simulink model "Problem3_AutomaticTransmissionControl"  (R2020b)
settings: Solver=ode5  StartTime=0.0  StopTime=50  FixedStep=0.04  RelTol=1e-3
PreLoadFcn:
  | clearvars
  | load('vehicleData.mat')
StartFcn:
  | cput= cputime;
StopFcn:
  | disp("CPU Time Elapsed"); cputime-cput
undefined symbols (not defined in the file): DOWN_TABLE, DOWN_TH_BP, EMAP, Iei, Iv, Kfactor, N20, NE_VEC, Rfd, rload0, rload2, Rw, sigbuilder_block, speedratio, TH_VEC, Torkratio, UP_TABLE, UP_TH_BP
CloseFcn:
  | clearvars
settings Model: DataDictionary=Data.sldd  Creator=vigne  LastModifiedBy=prabhudevmaddipudi

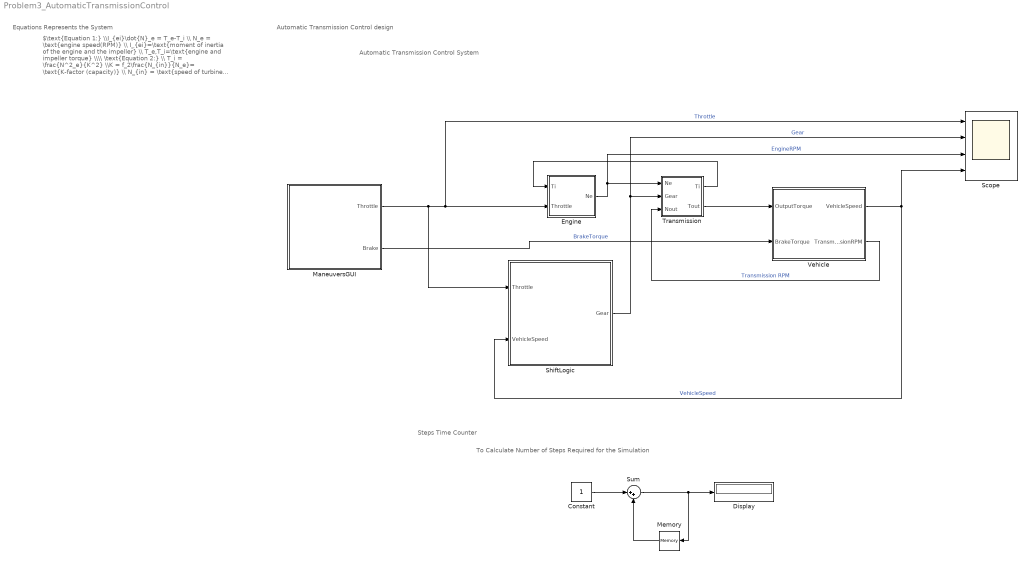
== system Problem3_AutomaticTransmissionControl ==
  note: Equations Represents the System
  note: $\text{Equation 1:} \\I_{ei}\dot{N}_e = T_e-T_i \\ N_e = \text{engine speed(RPM)} \\ I_{ei}=\text{moment of inertia of the engine and the impeller} \\ T_e,T_i=\text{engine and impeller torque} \\\\ \text{Equation 2:} \\ T_i = \frac{N^2_e}{K^2} \\K = f_2\frac{N_{in}}{N_e}= \text{K-factor (capacity)} \\ N_{in} = \text{speed of turbine (torque converter output)} \\ R_{TQ}= f_3\frac{N_{in}}{N_e}= \text{torque ratio} \\\\ \text{Equation 3:} \\ R_{TR}= f_4(gear) = \text{transmission ratio} \\ T_{out}=R_{TR}T_{in} \\ N_{in} = R_{TR}N_{out} \\ T_{in}, T_{out}= \text{transmission input and output torques} \\ N_{in}, N_{out} = \text{transmission input and output speed (RPM)} \\\\ \text{Equation 4:} \\ I_v\dot{N}_w= R_{fd}(T_{out}-T_{load}) \\ I_v= \text{vehicle inertia} \\ N_w = \text{wheel speed(RPM)} \\ R_{fd}= \text{final drive ratio} \\ T_{load}=f_s(N_w)=\text{load torque} \\\\ \text{Equation 5:} \\ T_{load}=sgn\left(mph\right)\left(R_{load0}+R_{load2}mph^2+T_{brake}\right) \\ R_{load0},R_{load2}= \text{friction and aerodynamic drag coefficients} \\ T_{load},T_{brake} = \text{load and break torque} \\ mph = \text{vehicle linear velocity}$
  note: Automatic Transmission Control design
  note: Steps Time Counter
  note: To Calculate Number of Steps Required for the Simulation
  note: Automatic Transmission Control System
  Constant : Constant
  Display : Display
  Engine : Subsystem
  ManeuversGUI : Subsystem  Tag=STV Subsys  LoadFcn=sigbuilder_block('load');  StartFcn=sigbuilder_block('start');  StopFcn=sigbuilder_block('stop');  ClipboardFcn=sigbuilder_block('clipboard');  mask(Sigbuilder block){tuvar=[0:10]}
      mask help: Sigbuilder GUI
      mask init:
      | tuvar = sigbuilder_block('maskInit');
      settings: CopyFcn=sigbuilder_block('copy');  DeleteFcn=sigbuilder_block('delete');  ModelCloseFcn=sigbuilder_block('modelClose');  PreSaveFcn=sigbuilder_block('preSave');  PauseFcn=sigbuilder_block('pause')  ContinueFcn=sigbuilder_block('continue')  NameChangeFcn=sigbuilder_block('namechange');  OpenFcn=sigbuilder_block('open',[6 22.5 1012.5 455.25 ]);  CloseFcn=sigbuilder_block('close');
      mask Display: plot(0, 0, 100, 100,[2, 2, 32, 32, 2], [68, 8, 8, 68, 68],[32, 2], [38, 38], [32, 19, 2],[53, 60, 44], [32, 17, 17, 2],[16, 16, 31, 31]);txt = getActiveGroup(gcbh);text(2, 100, txt,'verticalAlignment', 'top');
  Memory : Memory
  Scope : Scope  NumInputPorts=4
  ShiftLogic : Stateflow chart  TreatAsAtomicUnit=on
  Sum : Sum  Inputs=|++
  Transmission : Subsystem
  Vehicle : Subsystem
  wires:
  Transmission/2(Tout) -> Vehicle/1(OutputTorque)
  Transmission/1(Ti) -> Engine/1(Ti)
  Engine/1(Ne) -> Scope/3, Transmission/1(Ne)  "EngineRPM"
  ManeuversGUI/1(Throttle) -> ShiftLogic/1(Throttle), Scope/1, Engine/2(Throttle)  "Throttle"
  Vehicle/1(VehicleSpeed) -> Scope/4, ShiftLogic/2(VehicleSpeed)  "VehicleSpeed"
  Vehicle/2(TransmissionRPM) -> Transmission/3(Nout)  "Transmission RPM"
  ManeuversGUI/2(Brake) -> Vehicle/2(BrakeTorque)  "BrakeTorque"
  ShiftLogic/1(Gear) -> Scope/2, Transmission/2(Gear)  "Gear"
  Constant/1 -> Sum/1
  Sum/1 -> Memory/1, Display/1
  Memory/1 -> Sum/2

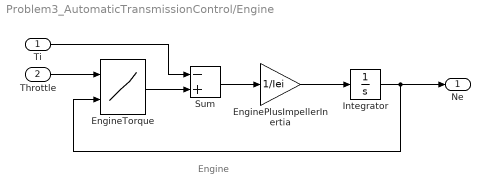
== system Problem3_AutomaticTransmissionControl/Engine ==
  note: Engine
  Ti : Inport  Unit=ft*lbf@torque
  Throttle : Inport  Port=2  Unit=%
  EnginePlusImpellerInertia : Gain  Gain=1/Iei  SaturateOnIntegerOverflow=on  OutDataTypeStr=Inherit: Same as input  ParamDataTypeStr=Inherit: Same as input
  EngineTorque : Lookup_n-D  BreakpointsForDimension1=TH_VEC  BreakpointsForDimension2=NE_VEC  Table=EMAP  InputSameDT=on
      settings: InputPortMap=u0,u1
  Integrator : Integrator  InitialCondition=1000  LimitOutput=on  UpperSaturationLimit=6000  LowerSaturationLimit=600  ZeroCross=off
  Sum : Sum  Inputs=-+  InputSameDT=on  SaturateOnIntegerOverflow=on  OutDataTypeStr=Inherit: Same as first input
  Ne : Outport  Unit=rpm  VectorParamsAs1DForOutWhenUnconnected=off
  wires:
  EnginePlusImpellerInertia/1 -> Integrator/1
  EngineTorque/1 -> Sum/2
  Ti/1 -> Sum/1
  Integrator/1 -> EngineTorque/2, Ne/1
  Throttle/1 -> EngineTorque/1
  Sum/1 -> EnginePlusImpellerInertia/1

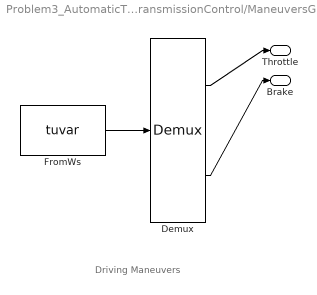
== system Problem3_AutomaticTransmissionControl/ManeuversGUI ==
  note: Driving Maneuvers
  Demux : Demux  Tag=STV Demux  Outputs=2
      settings: DisplayOption=none
  FromWs : FromWorkspace  Tag=STV FromWs  VariableName=tuvar  ZeroCross=off
      SigBuilderData=|
      | dataSet(1).timeRange = [0 50]
      | dataSet(1).name = 'Passing Maneuver'
      | dataSet(2).timeRange = [0 50]
      | dataSet(2).name = 'Gradual Acceleration'
      | dataSet(3).timeRange = [0 50]
      | dataSet(3).name = 'Hard braking'
      | dataSet(4).timeRange = [0 50]
      | dataSet(4).name = 'Coasting'
      | sbobj.Groups(1).Name = 'Passing Maneuver'
      | sbobj.Groups(1).Signals(1).Name = 'Throttle'
      | sbobj.Groups(1).Signals(1).XData = [0 14.9 15 27.55 33.45 40 50]
      | sbobj.Groups(1).Signals(1).YData = [60 40 100 1 80 41 100]
      | sbobj.Groups(1).Signals(2).Name = 'Brake'
      | sbobj.Groups(1).Signals(2).XData = [0 44.95 44.95 50]
      | sbobj.Groups(1).Signals(2).YData = [0 0 -0.55 -0.55]
      | sbobj.Groups(1).TimeRange = [0 50]
      | sbobj.Groups(2).Name = 'Gradual Acceleration'
      | sbobj.Groups(2).Signals(1).Name = 'Throttle'
      | sbobj.Groups(2).Signals(1).XData = [0 50]
      | sbobj.Groups(2).Signals(1).YData = [13.4 24]
      | sbobj.Groups(2).Signals(2).Name = 'Brake'
      | sbobj.Groups(2).Signals(2).XData = [0 50]
      | sbobj.Groups(2).Signals(2).YData = [0 0]
      | sbobj.Groups(2).TimeRange = [0 50]
      | sbobj.Groups(3).Name = 'Hard braking'
      | sbobj.Groups(3).Signals(1).Name = 'Throttle'
      | sbobj.Groups(3).Signals(1).XData = [0 5.1 5.1 50]
      | sbobj.Groups(3).Signals(1).YData = [50 50 1 1]
      | sbobj.Groups(3).Signals(2).Name = 'Brake'
      | sbobj.Groups(3).Signals(2).XData = [0 10 10 50]
      | sbobj.Groups(3).Signals(2).YData = [0 0 325 325]
      | sbobj.Groups(3).TimeRange = [0 50]
      | sbobj.Groups(4).Name = 'Coasting'
      | sbobj.Groups(4).Signals(1).Name = 'Throttle'
      | sbobj.Groups(4).Signals(1).XData = [0 4.8 4.8 50]
      | sbobj.Groups(4).Signals(1).YData = [80 80 1 1]
      | sbobj.Groups(4).Signals(2).Name = 'Brake'
      | sbobj.Groups(4).Signals(2).XData = [0 50]
      | sbobj.Groups(4).Signals(2).YData = [0 0]
      | sbobj.Groups(4).TimeRange = [0 50]
  Throttle : Outport  Tag=STV Outport  VectorParamsAs1DForOutWhenUnconnected=off
  Brake : Outport  Tag=STV Outport  Port=2  VectorParamsAs1DForOutWhenUnconnected=off
  wires:
  FromWs/1 -> Demux/1
  Demux/1 -> Throttle/1
  Demux/2 -> Brake/1

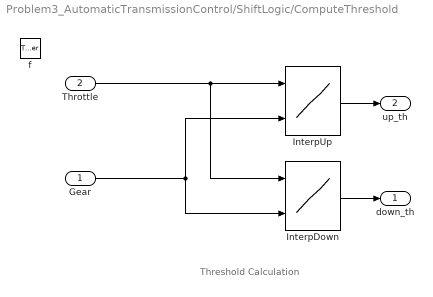
== system Problem3_AutomaticTransmissionControl/ShiftLogic/ComputeThreshold ==
  note: Threshold Calculation
  Gear : Inport
  Throttle : Inport  Port=2
  f : TriggerPort  TriggerType=function-call  VariantControl=(inherit)
      settings: CopyFcn=Stateflow.SLINSF.SimulinkMan.removeBlockPreDeleteFcn  PreDeleteFcn=Stateflow.SLINSF.SimulinkMan.unsafePredeleteFcn
  InterpDown : Lookup_n-D  BreakpointsForDimension1=DOWN_TH_BP  BreakpointsForDimension2=[1:4]  Table=DOWN_TABLE  OutDataTypeStr=double  LockScale=on
      settings: InputPortMap=u0,u1
  InterpUp : Lookup_n-D  BreakpointsForDimension1=UP_TH_BP  BreakpointsForDimension2=[1:4]  Table=UP_TABLE  OutDataTypeStr=double  LockScale=on
      settings: InputPortMap=u0,u1
  down_th : Outport  InitialOutput=0  VectorParamsAs1DForOutWhenUnconnected=off
  up_th : Outport  Port=2  InitialOutput=0  VectorParamsAs1DForOutWhenUnconnected=off
  wires:
  InterpUp/1 -> up_th/1
  InterpDown/1 -> down_th/1
  Throttle/1 -> InterpDown/1, InterpUp/1
  Gear/1 -> InterpDown/2, InterpUp/2

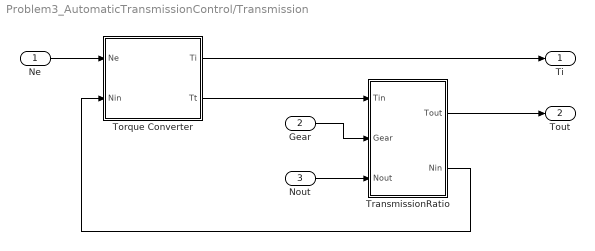
== system Problem3_AutomaticTransmissionControl/Transmission ==
  Ne : Inport  Unit=rpm
  Gear : Inport  Port=2  Unit=1
  Nout : Inport  Port=3  Unit=rpm
  Torque Converter : Subsystem
  TransmissionRatio : Subsystem
  Ti : Outport  Unit=ft*lbf@torque  VectorParamsAs1DForOutWhenUnconnected=off
  Tout : Outport  Port=2  Unit=ft*lbf@torque  VectorParamsAs1DForOutWhenUnconnected=off
  wires:
  Torque Converter/2(Tt) -> TransmissionRatio/1(Tin)
  Ne/1 -> Torque Converter/1(Ne)
  Torque Converter/1(Ti) -> Ti/1
  Nout/1 -> TransmissionRatio/3(Nout)
  Gear/1 -> TransmissionRatio/2(Gear)
  TransmissionRatio/2(Nin) -> Torque Converter/2(Nin)
  TransmissionRatio/1(Tout) -> Tout/1

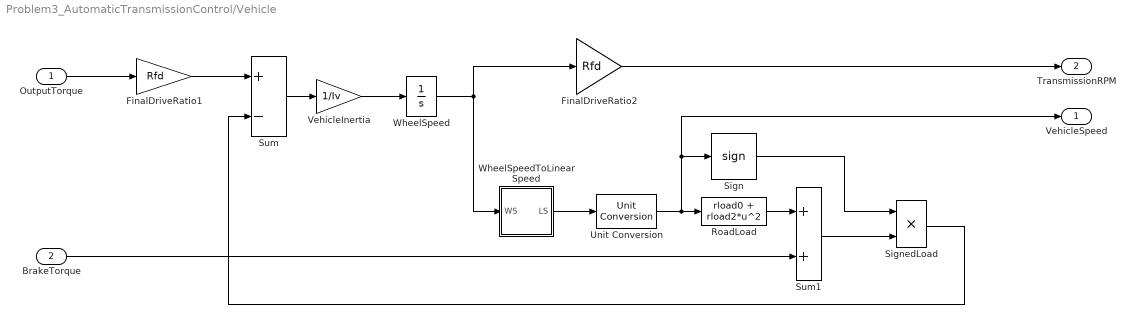
== system Problem3_AutomaticTransmissionControl/Vehicle ==
  OutputTorque : Inport  Unit=ft*lbf@torque
  BrakeTorque : Inport  Port=2  Unit=ft*lbf@torque
  FinalDriveRatio1 : Gain  Gain=Rfd  SaturateOnIntegerOverflow=on  OutDataTypeStr=Inherit: Same as input  ParamDataTypeStr=Inherit: Same as input
  FinalDriveRatio2 : Gain  Gain=Rfd  SaturateOnIntegerOverflow=on  OutDataTypeStr=Inherit: Same as input  ParamDataTypeStr=Inherit: Same as input
  RoadLoad : Fcn  Expr=rload0 + rload2*u^2
  Sign : Signum
  SignedLoad : Product  InputSameDT=on  SaturateOnIntegerOverflow=on  OutDataTypeStr=Inherit: Same as first input
  Sum : Sum  Inputs=+-  InputSameDT=on  SaturateOnIntegerOverflow=on  OutDataTypeStr=Inherit: Same as first input
  Sum1 : Sum  InputSameDT=on  SaturateOnIntegerOverflow=on  OutDataTypeStr=Inherit: Same as first input
  Unit Conversion : UnitConversion
  VehicleInertia : Gain  Gain=1/Iv  SaturateOnIntegerOverflow=on  OutDataTypeStr=Inherit: Same as input  ParamDataTypeStr=Inherit: Same as input
  WheelSpeed : Integrator  InitialCondition=N20/Rfd  ZeroCross=off
  WheelSpeedToLinearSpeed : Subsystem
  VehicleSpeed : Outport  Unit=mph  VectorParamsAs1DForOutWhenUnconnected=off
  TransmissionRPM : Outport  Port=2  Unit=rpm  VectorParamsAs1DForOutWhenUnconnected=off
  wires:
  FinalDriveRatio2/1 -> TransmissionRPM/1
  Unit Conversion/1 -> VehicleSpeed/1, Sign/1, RoadLoad/1
  OutputTorque/1 -> FinalDriveRatio1/1
  Sum1/1 -> SignedLoad/2
  WheelSpeed/1 -> FinalDriveRatio2/1, WheelSpeedToLinearSpeed/1(WS)
  WheelSpeedToLinearSpeed/1(LS) -> Unit Conversion/1
  Sum/1 -> VehicleInertia/1
  Sign/1 -> SignedLoad/1
  BrakeTorque/1 -> Sum1/2
  SignedLoad/1 -> Sum/2
  RoadLoad/1 -> Sum1/1
  VehicleInertia/1 -> WheelSpeed/1
  FinalDriveRatio1/1 -> Sum/1

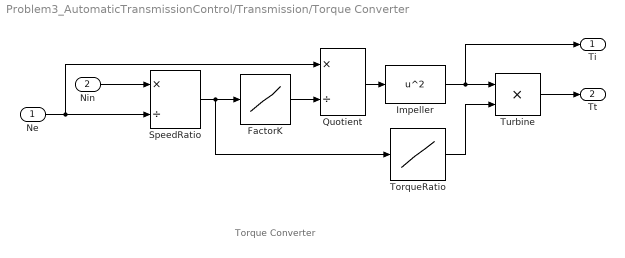
== system Problem3_AutomaticTransmissionControl/Transmission/Torque Converter ==
  note: Torque Converter
  Ne : Inport
  Nin : Inport  Port=2
  FactorK : Lookup_n-D  NumberOfTableDimensions=1  BreakpointsForDimension1=speedratio  Table=Kfactor  SaturateOnIntegerOverflow=on  InputSameDT=on
  Impeller : Fcn  Expr=u^2
  Quotient : Product  Inputs=*/  InputSameDT=on  SaturateOnIntegerOverflow=on  OutDataTypeStr=Inherit: Same as first input
  SpeedRatio : Product  Inputs=*/  InputSameDT=on  SaturateOnIntegerOverflow=on  OutDataTypeStr=Inherit: Same as first input
  TorqueRatio : Lookup_n-D  NumberOfTableDimensions=1  BreakpointsForDimension1=speedratio  Table=Torkratio  SaturateOnIntegerOverflow=on  InputSameDT=on
  Turbine : Product  InputSameDT=on  SaturateOnIntegerOverflow=on  OutDataTypeStr=Inherit: Same as first input
  Ti : Outport  VectorParamsAs1DForOutWhenUnconnected=off
  Tt : Outport  Port=2  VectorParamsAs1DForOutWhenUnconnected=off
  wires:
  Quotient/1 -> Impeller/1
  TorqueRatio/1 -> Turbine/2
  FactorK/1 -> Quotient/2
  Ne/1 -> SpeedRatio/2, Quotient/1
  Nin/1 -> SpeedRatio/1
  SpeedRatio/1 -> TorqueRatio/1, FactorK/1
  Impeller/1 -> Ti/1, Turbine/1
  Turbine/1 -> Tt/1

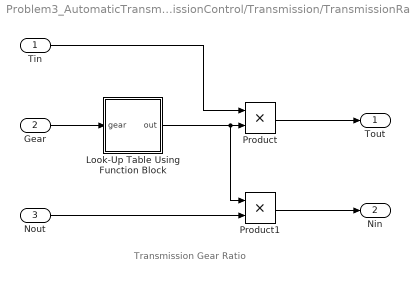
== system Problem3_AutomaticTransmissionControl/Transmission/TransmissionRatio ==
  note: Transmission Gear Ratio
  Tin : Inport  Unit=ft*lbf@torque
  Gear : Inport  Port=2  Unit=1
  Nout : Inport  Port=3  Unit=rpm
  Look-Up Table Using Function Block : MATLAB Function  TreatAsAtomicUnit=on
  Product : Product  InputSameDT=on  SaturateOnIntegerOverflow=on  OutDataTypeStr=Inherit: Same as first input
  Product1 : Product  InputSameDT=on  SaturateOnIntegerOverflow=on  OutDataTypeStr=Inherit: Same as first input
  Tout : Outport  Unit=ft*lbf@torque  VectorParamsAs1DForOutWhenUnconnected=off
  Nin : Outport  Port=2  Unit=rpm  VectorParamsAs1DForOutWhenUnconnected=off
  wires:
  Nout/1 -> Product1/2
  Look-Up Table Using Function Block/1(out) -> Product1/1, Product/2
  Product1/1 -> Nin/1
  Gear/1 -> Look-Up Table Using Function Block/1(gear)
  Tin/1 -> Product/1
  Product/1 -> Tout/1

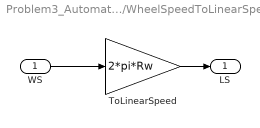
== system Problem3_AutomaticTransmissionControl/Vehicle/WheelSpeedToLinearSpeed ==
  WS : Inport  Unit=rpm
  ToLinearSpeed : Gain  Gain=2*pi*Rw  SaturateOnIntegerOverflow=on  OutDataTypeStr=Inherit: Same as input  ParamDataTypeStr=Inherit: Same as input
  LS : Outport  Unit=ft/min  VectorParamsAs1DForOutWhenUnconnected=off
  wires:
  ToLinearSpeed/1 -> LS/1
  WS/1 -> ToLinearSpeed/1

== stateflow chart Problem3_AutomaticTransmissionControl/ShiftLogic ==
  settings: updateMethod=DISCRETE  sampleTime=0.04
  state gear_state [parallel]
    settings: executionOrder=1
    state first
      entry:
      Gear = 1;
    state second
      entry:
      Gear = 2;
    state third
      entry:
      Gear = 3;
    state fourth
      entry:
      Gear = 4;
    (default) -> first
    second -> first [order 1] : DOWN
    first -> second : UP
    third -> second [order 1] : DOWN
    second -> third [order 2] : UP
    fourth -> third : DOWN
    third -> fourth [order 2] : UP
  state selection_state [parallel]
    during:
    [down_th, up_th] = ComputeThreshold(Gear,Throttle);
    settings: executionOrder=2
    state steady_state
    state upshifting
    state downshifting
    (default) -> steady_state
    downshifting -> steady_state [order 1] : after(TWAIT,tick)
        | [VehicleSpeed <= down_th]
        | {gear_state.DOWN}
    downshifting -> steady_state [order 2] : [VehicleSpeed > down_th]
    steady_state -> downshifting [order 2] : [VehicleSpeed < down_th]
    upshifting -> steady_state [order 2] : [VehicleSpeed < up_th]
    steady_state -> upshifting [order 1] : [VehicleSpeed > up_th]
    upshifting -> steady_state [order 1] : after(TWAIT,tick)
        | [VehicleSpeed >= up_th]
        | {gear_state.UP}
  state [down_th,up_th] = ComputeThreshold(Gear,Throttle) [function]
  data: Gear function_input; Throttle function_input; down_th function_output; up_th function_output; Throttle input double; VehicleSpeed input double; Gear output fixdt(0,8,5) [1..4]; TWAIT parameter fixdt(0,8,6); down_th local double; up_th local double
  events: DOWN local EITHER_EDGE_EVENT; UP local EITHER_EDGE_EVENT

== matlab function Problem3_AutomaticTransmissionControl/Transmission/TransmissionRatio/Look-Up Table Using Function Block ==
  data: gear input; out output
function out = fcn(gear)
    %#codegen
    table = [2.393 1.450 1.000 0.677];
    switch(gear)
        case gearType.fourth
            out=table(4);        
        case gearType.third
            out=table(3);            
        case gearType.second
            out=table(2);
        otherwise % gearType.first
            out=table(1);
    end
    
end
